simulink model "CIC_decimator_HDL_model"  (R2018b)
settings: Solver=VariableStepAuto  StartTime=0.0  StopTime=10.0  RelTol=1e-3
values from neighbouring files (symbols this model uses):
  CLK_DECIMATION_FACTOR = 50    [CIC_decimation_with_comp.m]
  R = 80    [CIC_decimation.m]    (also in CIC_decimation_with_comp.m = 125)
libraries: hdlsllib x5, simulink x4, dsphdlfiltering x1
settings Model: Creator=MrGoshak  LastModifiedBy=MrGoshak
settings HardwareCC: ProdBitPerPointer=32  ProdBitPerSizeT=32  ProdBitPerPtrDiffT=32  ProdLargestAtomicFloat=None  ProdIntDivRoundTo=Undefined  ProdEndianess=Unspecified  ProdWordSize=32  ProdHWDeviceType=ASIC/FPGA->ASIC/FPGA  TargetBitPerPointer=64  TargetBitPerSizeT=64  TargetBitPerPtrDiffT=64  TargetLongLongMode=on  TargetIntDivRoundTo=Zero  TargetEndianess=LittleEndian  TargetWordSize=64  TargetHWDeviceType=Custom Processor->MATLAB Host Computer  ProdEqTarget=off

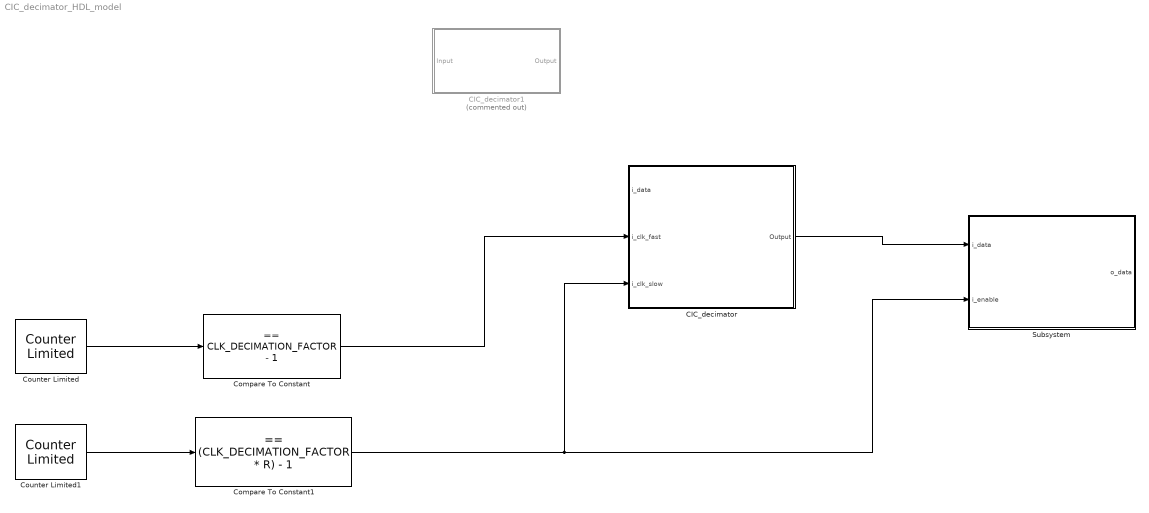
== system CIC_decimator_HDL_model ==
  CIC_decimator : Subsystem  Tag=FilterWizardSubSystem
      settings: ErrorFcn=dspFilterRealizedInBasicElemsAlgLoopErrFcnCallback
  CIC_decimator1 : Subsystem  Tag=FilterWizardSubSystem  Commented=on
      settings: ErrorFcn=dspFilterRealizedInBasicElemsAlgLoopErrFcnCallback
  Compare To Constant : simulink/Logic and Bit Operations/Compare To Constant  relop===  const=CLK_DECIMATION_FACTOR - 1  OutDataTypeStr=boolean
  Compare To Constant1 : simulink/Logic and Bit Operations/Compare To Constant  relop===  const=(CLK_DECIMATION_FACTOR * R) - 1  OutDataTypeStr=boolean
  Counter Limited : simulink/Sources/Counter Limited  uplimit=CLK_DECIMATION_FACTOR - 1  tsamp=-1
  Counter Limited1 : simulink/Sources/Counter Limited  uplimit=(CLK_DECIMATION_FACTOR * R) - 1  tsamp=-1
  Subsystem : Subsystem
  wires:
  Counter Limited/1 -> Compare To Constant/1
  Counter Limited1/1 -> Compare To Constant1/1
  Compare To Constant/1 -> CIC_decimator/2(i_clk_fast)
  Compare To Constant1/1 -> Subsystem/2(i_enable), CIC_decimator/3(i_clk_slow)
  CIC_decimator/1(Output) -> Subsystem/1(i_data)

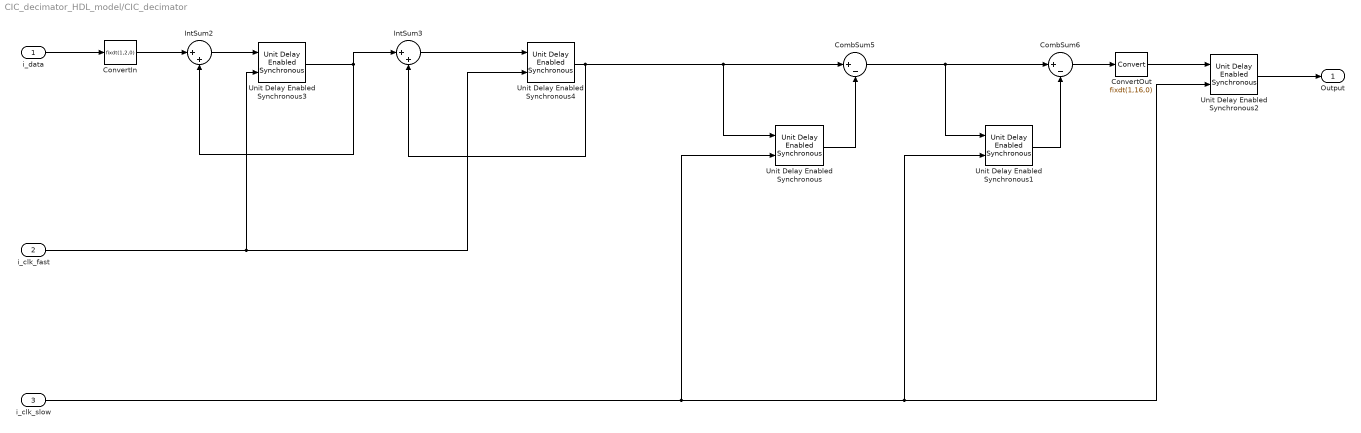
== system CIC_decimator_HDL_model/CIC_decimator ==
  i_data : Inport
  i_clk_fast : Inport  Port=2
  i_clk_slow : Inport  Port=3
  CombSum5 : Sum  Inputs=|+-  AccumDataTypeStr=fixdt(1,16,0)  OutDataTypeStr=fixdt(1,16,0)
  CombSum6 : Sum  Inputs=|+-  AccumDataTypeStr=fixdt(1,16,0)  OutDataTypeStr=fixdt(1,16,0)
  ConvertIn : DataTypeConversion  OutDataTypeStr=fixdt(1,2,0)  RndMeth=Nearest  SaturateOnIntegerOverflow=on
  ConvertOut : DataTypeConversion  OutDataTypeStr=fixdt(1,16,0)
  IntSum2 : Sum  Inputs=|++  AccumDataTypeStr=fixdt(1,16,0)  OutDataTypeStr=fixdt(1,16,0)
  IntSum3 : Sum  Inputs=|++  AccumDataTypeStr=fixdt(1,16,0)  OutDataTypeStr=fixdt(1,16,0)
  Unit Delay Enabled Synchronous{,1..4} (5 alike) : hdlsllib/Discrete/Unit Delay Enabled Synchronous  InitialCondition=0.0  SampleTime=-1
      settings: SourceProductName=HDL Coder  SourceProductBaseCode=HD
  Output : Outport
  wires:
  i_data/1 -> ConvertIn/1
  ConvertIn/1 -> IntSum2/1
  Unit Delay Enabled Synchronous3/1 -> IntSum2/2, IntSum3/1
  IntSum3/1 -> Unit Delay Enabled Synchronous4/1
  CombSum5/1 -> Unit Delay Enabled Synchronous1/1, CombSum6/1
  Unit Delay Enabled Synchronous/1 -> CombSum5/2
  Unit Delay Enabled Synchronous1/1 -> CombSum6/2
  CombSum6/1 -> ConvertOut/1
  ConvertOut/1 -> Unit Delay Enabled Synchronous2/1
  Unit Delay Enabled Synchronous2/1 -> Output/1
  IntSum2/1 -> Unit Delay Enabled Synchronous3/1
  Unit Delay Enabled Synchronous4/1 -> Unit Delay Enabled Synchronous/1, CombSum5/1, IntSum3/2
  i_clk_fast/1 -> Unit Delay Enabled Synchronous3/2, Unit Delay Enabled Synchronous4/2
  i_clk_slow/1 -> Unit Delay Enabled Synchronous1/2, Unit Delay Enabled Synchronous2/2, Unit Delay Enabled Synchronous/2

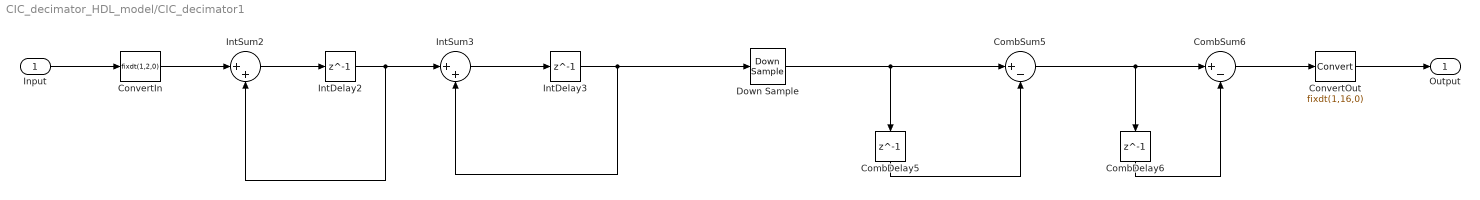
== system CIC_decimator_HDL_model/CIC_decimator1 ==
  Input : Inport
  CombDelay5 : Delay  DelayLength=1  InitialCondition=0
  CombDelay6 : Delay  DelayLength=1  InitialCondition=0
  CombSum5 : Sum  Inputs=|+-  AccumDataTypeStr=fixdt(1,16,0)  OutDataTypeStr=fixdt(1,16,0)
  CombSum6 : Sum  Inputs=|+-  AccumDataTypeStr=fixdt(1,16,0)  OutDataTypeStr=fixdt(1,16,0)
  ConvertIn : DataTypeConversion  OutDataTypeStr=fixdt(1,2,0)  RndMeth=Nearest  SaturateOnIntegerOverflow=on
  ConvertOut : DataTypeConversion  OutDataTypeStr=fixdt(1,16,0)
  Down Sample : DownSample  N=80  RateOptions=Allow multirate processing
  IntDelay2 : Delay  DelayLength=1  InitialCondition=0
  IntDelay3 : Delay  DelayLength=1  InitialCondition=0
  IntSum2 : Sum  Inputs=|++  AccumDataTypeStr=fixdt(1,16,0)  OutDataTypeStr=fixdt(1,16,0)
  IntSum3 : Sum  Inputs=|++  AccumDataTypeStr=fixdt(1,16,0)  OutDataTypeStr=fixdt(1,16,0)
  Output : Outport
  wires:
  Input/1 -> ConvertIn/1
  ConvertIn/1 -> IntSum2/1
  IntSum2/1 -> IntDelay2/1
  IntDelay2/1 -> IntSum2/2, IntSum3/1
  IntSum3/1 -> IntDelay3/1
  IntDelay3/1 -> IntSum3/2, Down Sample/1
  CombSum5/1 -> CombSum6/1, CombDelay6/1
  CombDelay5/1 -> CombSum5/2
  Down Sample/1 -> CombSum5/1, CombDelay5/1
  CombSum6/1 -> ConvertOut/1
  CombDelay6/1 -> CombSum6/2
  ConvertOut/1 -> Output/1

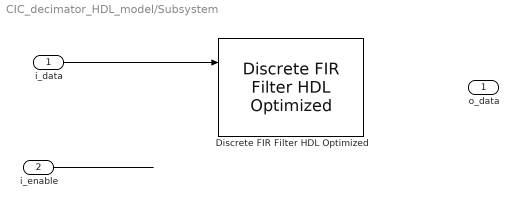
== system CIC_decimator_HDL_model/Subsystem ==
  i_data : Inport
  i_enable : Inport  Port=2
  Discrete FIR Filter HDL Optimized : dsphdlfiltering/Discrete FIR Filter HDL Optimized  Numerator=[ 0.5, 0.5 ]  FilterStructure=Direct form transposed  Sharing=off  SharingFactor=2  SimulateUsing=Code generation  roundingMode=Floor  overflowMode=off  CoefficientsDataTypeStr=Inherit: Same word length as input  CoefficientsMin=[]  CoefficientsMax=[]  OutputMin=[]  OutputMax=[]  ResetInputPort=off  HDLGlobalReset=on
      settings: SourceProductName=DSP System Toolbox  SourceProductBaseCode=DS
  o_data : Outport
  wires:
  i_data/1 -> Discrete FIR Filter HDL Optimized/1
  i_enable/1 -> ?
  ? -> o_data/1
